simulink model "xy_plot"  (R2018a)
settings: Solver=FixedStepAuto  StartTime=0.0  StopTime=10  FixedStep=0.01  RelTol=1e-3
libraries: instrumentlib x1, simulink x1
settings Model: Creator=U500304  LastModifiedBy=U500304

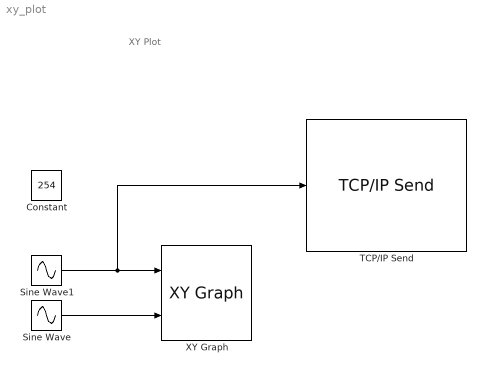
== system xy_plot ==
  note: XY Plot
  Constant : Constant  Value=254  SampleTime=0.1
  Sine Wave : Sin  Amplitude=5  SampleTime=0
  Sine Wave1 : Sin  Amplitude=2  Frequency=0.5  SampleTime=0.01
  TCP/IP Send : instrumentlib/TCP//IP Send  Host=localhost  Port=50000  EnableBlockingMode=on  Timeout=1  ByteOrder=BigEndian  TransferDelay=on
      settings: SourceProductName=Instrument Control Toolbox
  XY Graph : simulink/Sinks/XY Graph  xmin=-10  xmax=10  ymin=-10  ymax=10  st=-1
  wires:
  Sine Wave/1 -> XY Graph/2
  Sine Wave1/1 -> TCP/IP Send/1, XY Graph/1
